simulink model "Ex23"  (R2019b)
settings: Solver=VariableStepAuto  StartTime=0.0  StopTime=100.0  RelTol=1e-3
values from neighbouring files (symbols this model uses):
  D = D_v(i)    [Ex_10.m]    (also in Ex_20.m = 3000; Ex_22.m = 0.4; Ex_23.m = 0.1; Ex_29.m = 0.1)
  J = 0.4    [Ex_21.m]    (also in Ex_22.m = 1; Ex_23.m = 1.1; Ex_29.m = 1.1; Untitled2.m = 1)
  Kg = 0.1    [Ex_23.m]    (also in Ex_29.m)
  Km = 1    [Ex_23.m]    (also in Ex_29.m)
  L = 0.2    [Ex_23.m]    (also in Ex_27.m = 0.0001; Ex_29.m; Ex_8.m = 0.001; Ex_9.m = 0.001)
  R = 0.2    [Ex_21.m]    (also in Ex_22.m; Ex_23.m = 1.3; Ex_27.m = 2*qsi * sqrt(L/C); Ex_29.m = 1.3)
settings Model: Creator=andre  LastModifiedBy=andre

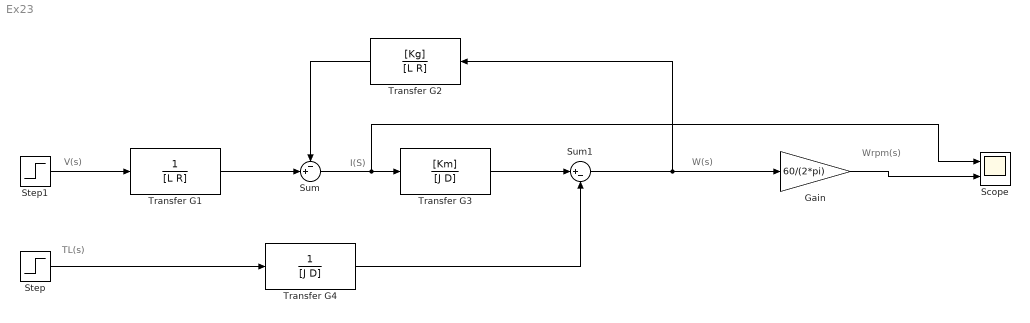
== system Ex23 ==
  note: Wrpm(s)
  note: W(s)
  note: I(S)
  note: TL(s)
  note: V(s)
  Gain : Gain  Gain=60/(2*pi)
  Scope : Scope  NumInputPorts=2
  Step : Step  Time=50  After=5  SampleTime=0
  Step1 : Step  Time=0  After=10  SampleTime=0
  Sum : Sum  Inputs=-+|
  Sum1 : Sum  Inputs=|+-
  Transfer G1 : TransferFcn  Denominator=[L R]
  Transfer G2 : TransferFcn  Numerator=[Kg]  Denominator=[L R]
  Transfer G3 : TransferFcn  Numerator=[Km]  Denominator=[J D]
  Transfer G4 : TransferFcn  Denominator=[J D]
  wires:
  Transfer G3/1 -> Sum1/1
  Sum/1 -> Scope/1, Transfer G3/1
  Transfer G4/1 -> Sum1/2
  Sum1/1 -> Gain/1, Transfer G2/1
  Transfer G1/1 -> Sum/2
  Transfer G2/1 -> Sum/1
  Step1/1 -> Transfer G1/1
  Step/1 -> Transfer G4/1
  Gain/1 -> Scope/2
